simulink library "PoolDelay"  (R2022b)
settings: Solver=VariableStepAuto  StartTime=0.0  StopTime=10.0  RelTol=1e-3
libraries: HandyTextFile x1
settings Model: Creator=ud1041536  LastModifiedBy=jk1043656
settings SolverCC: AlgebraicLoopSolver=TrustRegion
settings DataIOCC: ReturnWorkspaceOutputs=off
settings DebuggingCC: UnconnectedInputMsg=warning  UnconnectedOutputMsg=warning  UnconnectedLineMsg=warning  SFMachineParentedDataDiag=warning  ArithmeticOperatorsInVariantConditions=warning
settings ModelReferenceCC: EnableRefExpFcnMdlSchedulingChecks=on
settings SFSimCC: CustomCodeUndefinedFunction=UseInterfaceOnly

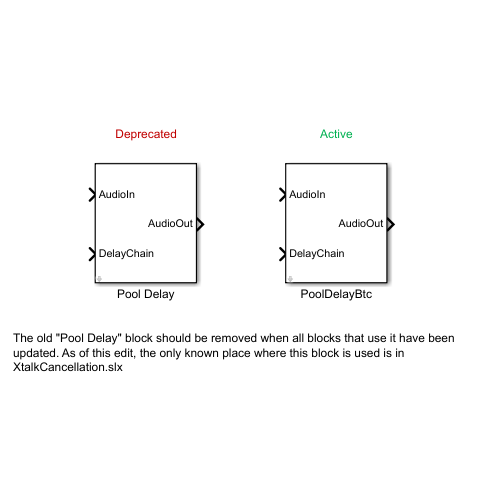
[thumbnail: Simulink's stored preview of the top-level diagram]
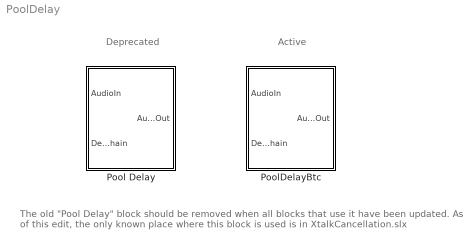
== system PoolDelay ==
  note: The old "Pool Delay" block should be removed when all blocks that use it have been updated. As of this edit, the only known place where this block is used is in XtalkCancellation.slx
  note: Deprecated
  note: Active
  Pool Delay : Subsystem  mask(Pool Delay){maxTotalDelay=512, frameSize=32, numChannels=2, bufferAlias=[], headerFilename=[]}
      mask prompts: maxTotalDelay "Total alloted delay"; frameSize "Frame size"; numChannels "Number of channels"; bufferAlias "Buffer alias"; headerFilename "Header file name"
      mask help:
      | Pool Delay is a multi-channel delay module with one single delay pool and adjustable delays per channel.
      |
      | Note: Please provide a Buffer Alias to the delay in order to access and edit the Header File Name.
      |
      | For more information, please see 'Help'.
      mask init:
      | blkh = gcbh;
      | MedusaDelayMaskInit(blkh, bufferAlias, headerFilename);
      mask Help:
      | Help on Mask Parameters:
      | 
      | Max Delay (in samples), Frame Size and Number of Channels help determine the circular buffer size. Buffer Alias and Header File Name are useful for memory management in cases where multiple delays are implemented. Both Buffer Alias and Header File Name are reflected in generated code.
      | 
      | Max Total Delay (in samples): Total alloted delay pool
      | Frame Size: Frame Size of the incoming audio
      | Number of Channels: Number of channels in incoming audio
      | Buffer Alias: Alias for the circular buffer allocated for this delay instance.
      | Header File Name: Name for header file that specifically manages the delays
      | 
      | For example, if the incoming audio consists of three channels, the input delay chain should be a 1x3 matrix (e.g. [10 20 30]).
      | Each element of delay shall be applied to the corresponding channel fo incoming audio. In the above example, the first input channel would be delayed by 10 samples, the second channel by 20 samples and the third by 30 samples.
      mask Callback bufferAlias:
      | % Get the mask parameter values. This is a cell
      | % array of character vectors.
      | maskStr = get_param(gcb,'bufferAlias');
      | 
      | % Check the value of 'bufferalias'
      | if ~(strcmp(maskStr,"[]"))
      |     % Set the visibility of all parameters on when
      |     set_param(gcb,'MaskVisibilities',{'on';'on';'on';'on';'on'});
      | else
      |     % Turn off the visibility of the 'headerfilename' field
      |     set_param(gcb,'MaskVisibilities',{'on';'on';'on';'on';'off'});
      | end
      | 
      | % Check if the 'bufferAlias' field is empty
      | if isempty(maskStr)
      |     % Turn off the visibility of the 'headerfilename' field
      |     set_param(gcb,'MaskVisibilities',{'on';'on';'on';'on';'off'});
      |     % Default the value of 'bufferAlias'
      |     set_param(gcb,'bufferAlias',"[]");
      | end
  PoolDelayBtc : Subsystem  mask(Pool Delay){Config=[]}
      mask prompts: Config "PoolDelayBtcConfig"
      mask help:
      | Pool Delay is a multi-channel delay module with one single delay pool and adjustable delays per channel.
      |
      | Note: Please provide a Buffer Alias to the delay in order to access and edit the Header File Name.
      |
      | For more information, please see 'Help'.
      mask init:
      | blkh=gcbh;
      | Config=BTConfig.Assert(blkh,Config);
      | 
      | Config.Validate();
      | Config.DoMaskInit(blkh);
      mask Help:
      | Help on Mask Parameters:
      | 
      | Max Delay (in samples), Frame Size and Number of Channels help determine the circular buffer size. Buffer Alias and Header File Name are useful for memory management in cases where multiple delays are implemented. Both Buffer Alias and Header File Name are reflected in generated code.
      | 
      | Max Total Delay (in samples): Total alloted delay pool
      | Frame Size: Frame Size of the incoming audio
      | Number of Channels: Number of channels in incoming audio
      | Buffer Alias: Alias for the circular buffer allocated for this delay instance.
      | Header File Name: Name for header file that specifically manages the delays
      | 
      | For example, if the incoming audio consists of three channels, the input delay chain should be a 1x3 matrix (e.g. [10 20 30]).
      | Each element of delay shall be applied to the corresponding channel fo incoming audio. In the above example, the first input channel would be delayed by 10 samples, the second channel by 20 samples and the third by 30 samples.

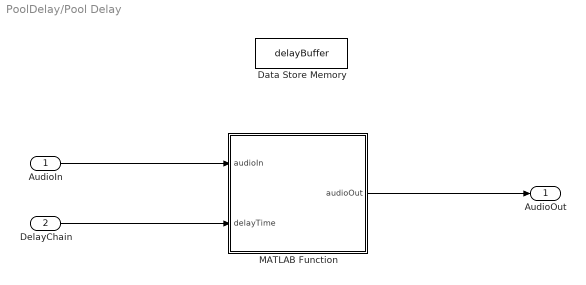
== system PoolDelay/Pool Delay ==
  AudioIn : Inport
  DelayChain : Inport  Port=2
  Data Store Memory : DataStoreMemory  DataStoreName=delayBuffer  ReadBeforeWriteMsg=warning  WriteAfterWriteMsg=warning  WriteAfterReadMsg=warning  InitialValue=zeros(maxTotalDelay,1)  ShowAdditionalParam=off  OutDataTypeStr=single
  MATLAB Function : MATLAB Function  TreatAsAtomicUnit=on
  AudioOut : Outport  VectorParamsAs1DForOutWhenUnconnected=off
  wires:
  DelayChain/1 -> MATLAB Function/2(delayTime)
  AudioIn/1 -> MATLAB Function/1(audioIn)
  MATLAB Function/1(audioOut) -> AudioOut/1

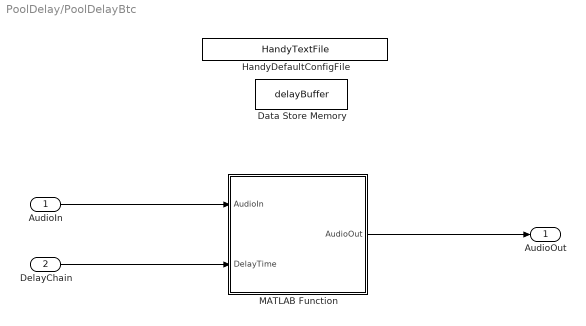
== system PoolDelay/PoolDelayBtc ==
  AudioIn : Inport
  DelayChain : Inport  Port=2
  Data Store Memory : DataStoreMemory  DataStoreName=delayBuffer  ReadBeforeWriteMsg=warning  WriteAfterWriteMsg=warning  WriteAfterReadMsg=warning  InitialValue=zeros(Config.MaxDelay,1)  ShowAdditionalParam=off  OutDataTypeStr=single
  HandyDefaultConfigFile : HandyTextFile/HandyTextFile  TemplateSource=Config  FileSuffix=Init  OpenDialogOnLoad=off  UseThisBlockName=off  TheDefaultText=|  ShowInLibBrowser=on
      | % $(FILENAME) Setup model parameters for each "Init" callback (e.g. update diagram)
      | sample_rate_in_hertz = 44100;
      | frame_size = 32;
      | sysin_channel_count = 2;
      settings: SourceProductName=Bose Talaria
  MATLAB Function : MATLAB Function  TreatAsAtomicUnit=on  mask{MaxDelay=Config.MaxDelay}
  AudioOut : Outport  VectorParamsAs1DForOutWhenUnconnected=off
  wires:
  DelayChain/1 -> MATLAB Function/2(DelayTime)
  AudioIn/1 -> MATLAB Function/1(AudioIn)
  MATLAB Function/1(AudioOut) -> AudioOut/1

== matlab function PoolDelay/PoolDelayBtc/MATLAB Function ==
  data: AudioIn input; AudioOut output; DelayTime input; MaxDelay parameter size=1; delayBuffer data_store_memory
function AudioOut = delay(AudioIn, DelayTime, MaxDelay)
%[param:MaxDelay]

% Our delayline lives in global variable. We treat as a circular buffer. 
global delayBuffer

% figure out the frame size and channel count
[frameSize, numChannels] = size(AudioIn);
frameSize = int32(frameSize);
MaxDelay = int32(MaxDelay);
AudioOut = coder.nullcopy(AudioIn);

% writeIndex points to our current write location in buffer
persistent delayIndex;
if isempty(delayIndex)
    delayIndex = int32(0);
end

bufferIndex = delayIndex;

% OUTPUT
for channel = 1:numChannels
    % Delay for current channel
    delay = DelayTime(channel); 
    
    % Number of samples into the delay buffer
    partialDelay = min(frameSize, delay);
    
    % Initial offset into delay buffer
    srcIndex = circindex(bufferIndex, int32(1), MaxDelay);
    
    % Fill first part of output buffer from delay buffer
    for sample = 1:partialDelay
        AudioOut(sample, channel) = delayBuffer(srcIndex + 1);
        srcIndex = circindex(srcIndex, int32(1), MaxDelay);
    end
    
    % Fill the rest from the input buffer
    for sample = partialDelay+1:frameSize
        AudioOut(sample, channel) = AudioIn(sample - partialDelay, channel);
    end
    
    % Advance buffer index for next channel
    bufferIndex = circindex(bufferIndex, delay, MaxDelay); 
end

% Reset and advance by one frame
bufferIndex = circindex(delayIndex, min(frameSize, MaxDelay), MaxDelay);
delayIndex = bufferIndex;

% DELAY LINE
for channel = 1:numChannels
    
    % Delay for current channel
    delay = DelayTime(channel); 
    
    % Number of samples into the delay buffer
    partialDelay = min(frameSize, delay);
    
    % Calculate index with offset
    destIndex = circindex(bufferIndex, delay - partialDelay + 1, MaxDelay);
    
    % Fill output buffer from delay buffer
    for sample = frameSize - partialDelay+1:frameSize
        delayBuffer(destIndex + 1) = AudioIn(sample, channel);
        destIndex = circindex(destIndex, int32(1), MaxDelay);
    end
    
    % Advance buffer index for next channel
    bufferIndex = circindex(bufferIndex, delay, MaxDelay); 
end

end

== matlab function PoolDelay/Pool Delay/MATLAB Function ==
  data: audioIn input; audioOut output; delayTime input; maxTotalDelay parameter size=1; delayBuffer data_store_memory
function audioOut = delay(audioIn, delayTime, maxTotalDelay)

% Our delayline lives in global variable. We treat as a circular buffer. 
global delayBuffer

% figure out the frame size and channel count
[frameSize, numChannels] = size(audioIn);
frameSize = int32(frameSize);
maxTotalDelay = int32(maxTotalDelay);
audioOut = coder.nullcopy(audioIn);

% writeIndex points to our current write location in buffer
persistent delayIndex;
if isempty(delayIndex)
    delayIndex = int32(0);
end

bufferIndex = delayIndex;

% OUTPUT
for channel = 1:numChannels
    % Delay for current channel
    delay = delayTime(channel); 
    
    % Number of samples into the delay buffer
    partialDelay = min(frameSize, delay);
    
    % Initial offset into delay buffer
    srcIndex = circindex(bufferIndex, int32(1), maxTotalDelay);
    
    % Fill first part of output buffer from delay buffer
    for sample = 1:partialDelay
        audioOut(sample, channel) = delayBuffer(srcIndex + 1);
        srcIndex = circindex(srcIndex, int32(1), maxTotalDelay);
    end
    
    % Fill the rest from the input buffer
    for sample = partialDelay+1:frameSize
        audioOut(sample, channel) = audioIn(sample - partialDelay, channel);
    end
    
    % Advance buffer index for next channel
    bufferIndex = circindex(bufferIndex, delay, maxTotalDelay); 
end

% Reset and advance by one frame
bufferIndex = circindex(delayIndex, min(frameSize, maxTotalDelay), maxTotalDelay);
delayIndex = bufferIndex;

% DELAY LINE
for channel = 1:numChannels
    
    % Delay for current channel
    delay = delayTime(channel); 
    
    % Number of samples into the delay buffer
    partialDelay = min(frameSize, delay);
    
    % Calculate index with offset
    destIndex = circindex(bufferIndex, delay - partialDelay + 1, maxTotalDelay);
    
    % Fill output buffer from delay buffer
    for sample = frameSize - partialDelay+1:frameSize
        delayBuffer(destIndex + 1) = audioIn(sample, channel);
        destIndex = circindex(destIndex, int32(1), maxTotalDelay);
    end
    
    % Advance buffer index for next channel
    bufferIndex = circindex(bufferIndex, delay, maxTotalDelay); 
end

end
